simulink model "TF"  (R2025a)
settings: Solver=VariableStepAuto  StartTime=0.0  StopTime=38.24  RelTol=1e-3
values from neighbouring files (symbols this model uses):
  Kd = gains(3)    [Experiment.m]
  Ki = gains(2)    [Experiment.m]
  Kp = gains(1)    [Experiment.m]
libraries: slpidlib x1
settings Model: Creator=Radit  LastModifiedBy=jeremyphilson

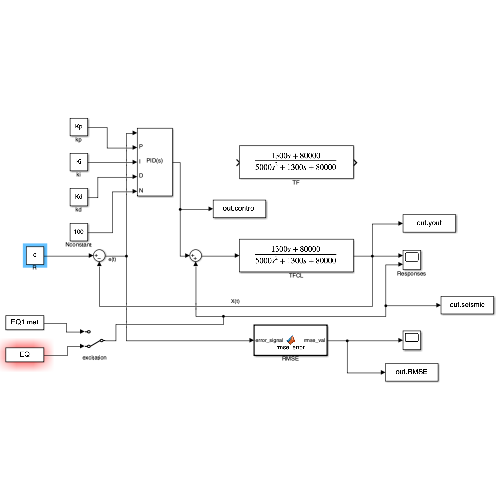
[thumbnail: Simulink's stored preview of the top-level diagram]
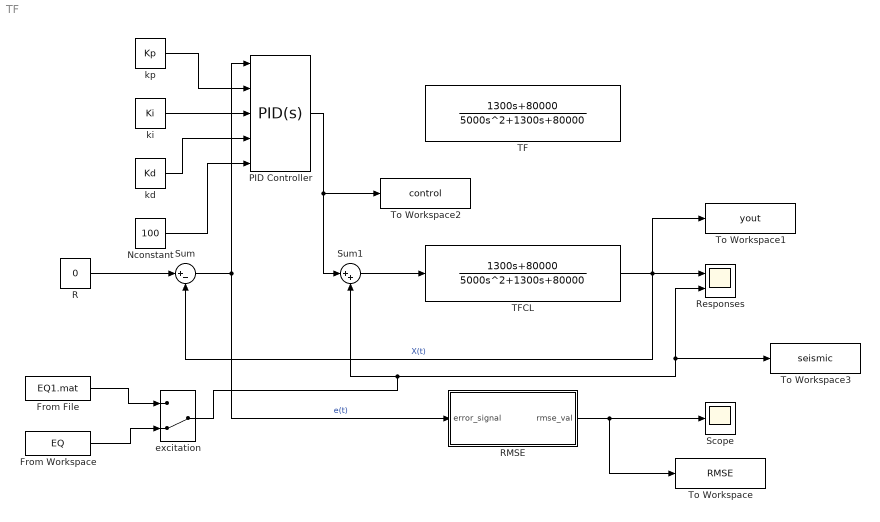
== system TF ==
  From Workspace : FromWorkspace  VariableName=EQ  OutputAfterFinalValue=Setting to zero
  From File : FromFile  FileName=EQ1.mat  SampleTime=0
  Nconstant : Constant  Value=100
  PID Controller : slpidlib/PID Controller  Controller=PID  Form=Parallel  TimeDomain=Continuous-time  UseExternalTs=off  SampleTime=-1  IntegratorMethod=Forward Euler  FilterMethod=Forward Euler  ControllerParametersSource=external  P=0  I=0  UseKiTs=off  D=0  UseExternalDerivativeSource=off  N=100  UseFilter=on  TunerSelectOption=Transfer Function Based (PID Tuner App)  InitialConditionSource=internal  InitialConditionForIntegrator=0  InitialConditionForFilter=0  DifferentiatorICPrevScaledInput=0  ExternalReset=none  TrackingMode=off  Kt=1  LimitOutput=off  SatLimitsSource=internal  UpperSaturationLimit=inf  LowerSaturationLimit=-inf  LinearizeAsGain=on  AntiWindupMode=none  Kb=1  LimitIntegrator=off  UpperIntegratorSaturationLimit=inf  LowerIntegratorSaturationLimit=-inf  POutMin=[]  POutMax=[]  IOutMin=[]  IOutMax=[]  DOutMin=[]  DOutMax=[]  NOutMin=[]  NOutMax=[]  SumOutMin=[]  SumOutMax=[]  SaturationOutMin=[]  SaturationOutMax=[]  PParamMin=[]  PParamMax=[]  IParamMin=[]  IParamMax=[]  DParamMin=[]  DParamMax=[]  NParamMin=[]  NParamMax=[]  KbParamMin=[]  KbParamMax=[]  KtParamMin=[]  KtParamMax=[]  KbOutMin=[]  KbOutMax=[]  KtOutMin=[]  KtOutMax=[]  IntegratorOutMin=[]  IntegratorOutMax=[]  FilterOutMin=[]  FilterOutMax=[]  SumI1OutMin=[]  SumI1OutMax=[]  SumI2OutMin=[]  SumI2OutMax=[]  SumI3OutMin=[]  SumI3OutMax=[]  SumI4OutMin=[]  SumI4OutMax=[]  SumDOutMin=[]  SumDOutMax=[]  DifferentiatorOutMin=[]  DifferentiatorOutMax=[]  FilterDiffOutCoefMin=[]  FilterDiffOutCoefMax=[]  ReciprocalOutMin=[]  ReciprocalOutMax=[]  SumDenOutMin=[]  SumDenOutMax=[]  SumNumOutMin=[]  SumNumOutMax=[]  DivideOutMin=[]  DivideOutMax=[]  UdiffTsProdOutMin=[]  UdiffTsProdOutMax=[]  NTsProdOutMin=[]  NTsProdOutMax=[]  UintegralTsProdOutMin=[]  UintegralTsProdOutMax=[]  UngainTsProdOutMin=[]  UngainTsProdOutMax=[]  ClampingZeroOutDataTypeStr=Inherit: Inherit via back propagation  ClampingZeroOutMin=[]  ClampingZeroOutMax=[]  FilterDenConstantOutDataTypeStr=Inherit: Inherit via back propagation  FilterDenConstantOutMin=[]  FilterDenConstantOutMax=[]  PCopyOutDataTypeStr=Inherit: Inherit via back propagation  PCopyOutMin=[]  PCopyOutMax=[]  NCopyOutDataTypeStr=Inherit: Inherit via back propagation  NCopyOutMin=[]  NCopyOutMax=[]  IntegratorContinuousStateAttributes=''  IntegratorStateMustResolveToSignalObject=off  IntegratorRTWStateStorageClass=Auto  FilterContinuousStateAttributes=''  FilterStateMustResolveToSignalObject=off  FilterRTWStateStorageClass=Auto  ParallelPVariant=ExternalParameters  IdealPVariant=Disabled  IVariant=ExternalParameters  DVariant=ExternalParameters  IntegratorVariant=Continuous  SatVariant=Disabled  AWVariant=Passthrough  PCopyVariant=Disabled  TRVariant=Disabled  FdbkBlocksVariant=Forward  IdealPFdbkVariant=Disabled  SatFdbkVariant=Disabled  DerivativeFilterVariant=ContFilter  NVariant=ExternalParameters  NCopyVariant=Disabled  FilterICVariant=InternalICsFilter  IntegratorICVariant=InternalICs  ExternalResetVariant=Disabled  TRSumVariant=Passthrough  SumFdbkVariant=Disabled  SumVariant=Sum_PID  TsampFilterVariant=InternalTs  TsampNgainVariant=Passthrough  TsampIntegralVariant=Disabled_SignalSpec  ExternalSaturationOutDataTypeStr=Inherit: Same as second input  DerivativeSourceVariant=ErrorSignal  PreIntVariant=InternalPreInt
  R : Constant  Value=0
  RMSE : MATLAB Function  TreatAsAtomicUnit=on
  Responses : Scope  NumInputPorts=2
      settings: ActiveDisplayYMinimum=-0.33843  ActiveDisplayYMaximum=0.42538
  Scope : Scope
      settings: ActiveDisplayYMinimum=-0.23133  ActiveDisplayYMaximum=2.08199
  Sum : Sum  Inputs=|+-
  Sum1 : Sum  Inputs=|++
  TF : TransferFcn  Numerator=[1300 80000]  Denominator=[5000 1300 80000]
  TFCL : TransferFcn  Numerator=[1300 80000]  Denominator=[5000 1300 80000]
  To Workspace : ToWorkspace  VariableName=RMSE  SaveFormat=Timeseries  SampleTime=-1
  To Workspace1 : ToWorkspace  VariableName=yout  SaveFormat=Timeseries  SampleTime=-1
  To Workspace2 : ToWorkspace  VariableName=control  SaveFormat=Timeseries  SampleTime=-1
  To Workspace3 : ToWorkspace  VariableName=seismic  SaveFormat=Timeseries  SampleTime=-1
  excitation : ManualSwitch  CurrentSetting=0
  kd : Constant  Value=Kd
  ki : Constant  Value=Ki
  kp : Constant  Value=Kp
  wires:
  TFCL/1 -> To Workspace1/1, Sum/2, Responses/1  "X(t)"
  R/1 -> Sum/1
  Sum1/1 -> TFCL/1
  PID Controller/1 -> Sum1/1, To Workspace2/1
  Sum/1 -> PID Controller/1, RMSE/1(error_signal)  "e(t)"
  Nconstant/1 -> PID Controller/5
  kp/1 -> PID Controller/2
  ki/1 -> PID Controller/3
  kd/1 -> PID Controller/4
  RMSE/1(rmse_val) -> To Workspace/1, Scope/1
  excitation/1 -> Sum1/2, To Workspace3/1, Responses/2
  From File/1 -> excitation/1
  From Workspace/1 -> excitation/2

== matlab function TF/RMSE ==
  data: error_signal input; rmse_val output
function rmse_val = rmse_error(error_signal)
    % pastikan dalam bentuk kolom
    %error_signal = error_signal(:);

    % komputasi RMSE
    rmse_val = sqrt( mean( error_signal.^2 ) );

end
